simulink model "sim_5_twolink_force_control"  (R2021a)
settings: Solver=VariableStepAuto  StartTime=0.0  StopTime=15  MaxStep=1e-2
values from neighbouring files (symbols this model uses):
  b1 = 0.01    [sim_params.m]    (also in sim_params_force.m)
  b2 = 0.01    [sim_params.m]    (also in sim_params_force.m)
  D = [zeros(n); eye(n)]    [control_comparison_script.m]    (also in gen_twolink_ss.m = reshape([0.0,0.0,0.0,0.0,0.0,0.0,0.0,0.0],[4,2]))
  g = 9.80665    [sim_params.m]    (also in sim_params_force.m)
  L1x = 0.3    [sim_params.m]    (also in sim_params_force.m)
  L1y = 0.050    (= 0.05)    [sim_params.m]    (also in sim_params_force.m)
  L1z = 0.05    [sim_params.m]    (also in sim_params_force.m)
  L2x = 0.15    [sim_params.m]    (also in sim_params_force.m = 0.3)
  L2y = 0.05    [sim_params.m]    (also in sim_params_force.m)
  L2z = 0.05    [sim_params.m]    (also in sim_params_force.m)
  m1 = m1*1.25    [control_comparison_script.m]    (also in sim_params.m = 2.775; sim_params_force.m = 2.775)
  m2 = m2*1.25    [control_comparison_script.m]    (also in sim_params.m = 1.3875; sim_params_force.m = 2.775)
  max_joint_torque1 = 20    [sim_params.m]    (also in sim_params_force.m)
  max_joint_torque2 = 10    [sim_params.m]    (also in sim_params_force.m = 20)
undefined symbols (not defined in the file or in its folder): Da, KD, KD_a, Kd_p, Kd_p2, Kdt, KF, Kf_v, Kf_v2, KI, Ki_f, Ki_f2, Ki_p, Ki_p2, KP, KP_a, Kp_f, Kp_f2, Kp_p, Kp_p2, Levenberg, Ma, Marquardt, R_env, sigbuilder_block, W_env, X, Xenv, Y, Z
libraries: sm_lib x72, nesl_utility x58, pid_lib x14, simulink x3, robotmaniplib x2, robotcorelib x1
(part 6 of 6)

== matlab function sim_5_twolink_force_control/Controller/Hybrid Force//position control /Position Controller1/Position Projection/Position projection (SJ)+ ==
  data: L_1 input; L_2 input; SJ_pinv output; theta_1 input; theta_2 input
function SJ_pinv = P_position(L_1,L_2,theta_1,theta_2)
% Position projection pinv(SJ)
% StJ_t = transpose((1-S)*J)

% position control in y axis
SJ_pinv = [
[0, (L_2*cos((theta_1))*L_1^2 + L_1*cos((theta_1) + (theta_2))*L_2^2)/(L_2^2*cos(theta_1 + theta_2)*L_1^2*cos((theta_1)) + L_1^2*cos(theta_1)*cos((theta_1) + (theta_2))*L_2^2 + L_1*L_2*cos(theta_1)*L_1^2*cos((theta_1)) + 2*L_1*L_2*cos((theta_1) + (theta_2))*cos(theta_1 + theta_2)*L_2^2)]
[0,                                        (L_1*cos((theta_1) + (theta_2))*L_2^2)/(L_2^2*cos(theta_1 + theta_2)*L_1^2*cos((theta_1)) + L_1^2*cos(theta_1)*cos((theta_1) + (theta_2))*L_2^2 + L_1*L_2*cos(theta_1)*L_1^2*cos(theta_1) + 2*L_1*L_2*cos(theta_1 + theta_2)*cos(theta_1 + theta_2)*L_2^2)]
];


% full position control 
% SJ_pinv = [
% [                                 cos(theta_1 + theta_2)/(L_1*sin(theta_2)),                                  sin(theta_1 + theta_2)/(L_1*sin(theta_2))]
% [-(L_2*cos(theta_1 + theta_2) + L_1*cos(theta_1))/(L_1*L_2*sin(theta_2)), -(L_1*sin(theta_1) + L_2*sin(theta_1 + theta_2))/(L_1*L_2*sin(theta_2))]
%     ];

== matlab function sim_5_twolink_force_control/Controller/Hybrid Force//position control /Position Controller1/Position Projection1/Position projection (SJ)+ ==
  data: L_1 input; L_2 input; SJ_pinv output; theta_1 input; theta_2 input
function SJ_pinv = P_position(L_1,L_2,theta_1,theta_2)
% Position projection pinv(SJ)
% StJ_t = transpose((1-S)*J)

% position control in y axis
SJ_pinv = [
[0, (L_2*cos((theta_1))*L_1^2 + L_1*cos((theta_1) + (theta_2))*L_2^2)/(L_2^2*cos(theta_1 + theta_2)*L_1^2*cos((theta_1)) + L_1^2*cos(theta_1)*cos((theta_1) + (theta_2))*L_2^2 + L_1*L_2*cos(theta_1)*L_1^2*cos((theta_1)) + 2*L_1*L_2*cos((theta_1) + (theta_2))*cos(theta_1 + theta_2)*L_2^2)]
[0,                                        (L_1*cos((theta_1) + (theta_2))*L_2^2)/(L_2^2*cos(theta_1 + theta_2)*L_1^2*cos((theta_1)) + L_1^2*cos(theta_1)*cos((theta_1) + (theta_2))*L_2^2 + L_1*L_2*cos(theta_1)*L_1^2*cos(theta_1) + 2*L_1*L_2*cos(theta_1 + theta_2)*cos(theta_1 + theta_2)*L_2^2)]
];


% full position control 
% SJ_pinv = [
% [                                 cos(theta_1 + theta_2)/(L_1*sin(theta_2)),                                  sin(theta_1 + theta_2)/(L_1*sin(theta_2))]
% [-(L_2*cos(theta_1 + theta_2) + L_1*cos(theta_1))/(L_1*L_2*sin(theta_2)), -(L_1*sin(theta_1) + L_2*sin(theta_1 + theta_2))/(L_1*L_2*sin(theta_2))]
%     ];

== matlab function sim_5_twolink_force_control/Controller/Hybrid Force//position control /Force Controller/Force Projection1/Force projection (StJ_t) ==
  data: L_1 input; L_2 input; StJ_t output; theta_1 input; theta_2 input
function StJ_t = P_force(L_1,L_2,theta_1,theta_2)
% Force projection (StJ_t)
% StJ_t = transpose((1-S)*J)

% force control in X axis
StJ_t = [
    [- L_1*sin(theta_1) - L_2*sin(theta_1 + theta_2), 0]
    [                    -L_2*sin(theta_1 + theta_2), 0]
];

% no force control at all

% StJ_t = [
%     0   0;
%     0   0;
% ];

== matlab function sim_5_twolink_force_control/Controller/Hybrid Force//position control /Force Controller/Force Projection2/Force projection (StJ_t) ==
  data: L_1 input; L_2 input; StJ_t output; theta_1 input; theta_2 input
function StJ_t = P_force(L_1,L_2,theta_1,theta_2)
% Force projection (StJ_t)
% StJ_t = transpose((1-S)*J)

% force control in X axis
StJ_t = [
    [- L_1*sin(theta_1) - L_2*sin(theta_1 + theta_2), 0]
    [                    -L_2*sin(theta_1 + theta_2), 0]
];

% no force control at all

% StJ_t = [
%     0   0;
%     0   0;
% ];

== matlab function sim_5_twolink_force_control/Controller/Hybrid Force//position control /Jacobian/Jacobian ==
  data: L_1 input; J output; L_2 input; theta_1 input; theta_2 input
function J = jacobian_geom(L_1,L_2,theta_1,theta_2)

J = [
       -L_1.*sin(theta_1)-L_2.*sin(theta_1+theta_2) , -L_2.*sin(theta_1+theta_2) ;
        L_1.*cos(theta_1)+L_2.*cos(theta_1+theta_2) ,  L_2.*cos(theta_1+theta_2) ;
    ];

== matlab function sim_5_twolink_force_control/Controller/Hybrid Force//position control (stiff)/Force Controller/Force Projection/Force projection (StJ_t) ==
  data: L_1 input; L_2 input; StJ_t output; theta_1 input; theta_2 input
function StJ_t = P_force(L_1,L_2,theta_1,theta_2)
% Force projection (StJ_t)
% StJ_t = transpose((1-S)*J)

% force control in X axis
StJ_t = [
    [- L_1*sin(theta_1) - L_2*sin(theta_1 + theta_2), 0]
    [                    -L_2*sin(theta_1 + theta_2), 0]
];

% no force control at all

% StJ_t = [
%     0   0;
%     0   0;
% ];

== matlab function sim_5_twolink_force_control/Controller/Hybrid Force//position control (stiff)/Force Controller/Force Projection1/Force projection (StJ_t) ==
  data: L_1 input; L_2 input; StJ_t output; theta_1 input; theta_2 input
function StJ_t = P_force(L_1,L_2,theta_1,theta_2)
% Force projection (StJ_t)
% StJ_t = transpose((1-S)*J)

% force control in X axis
StJ_t = [
    [- L_1*sin(theta_1) - L_2*sin(theta_1 + theta_2), 0]
    [                    -L_2*sin(theta_1 + theta_2), 0]
];

% no force control at all

% StJ_t = [
%     0   0;
%     0   0;
% ];

== matlab function sim_5_twolink_force_control/Controller/Hybrid Force//position control (stiff)/Force Controller/Force Projection2/Force projection (StJ_t) ==
  data: L_1 input; L_2 input; StJ_t output; theta_1 input; theta_2 input
function StJ_t = P_force(L_1,L_2,theta_1,theta_2)
% Force projection (StJ_t)
% StJ_t = transpose((1-S)*J)

% force control in X axis
StJ_t = [
    [- L_1*sin(theta_1) - L_2*sin(theta_1 + theta_2), 0]
    [                    -L_2*sin(theta_1 + theta_2), 0]
];

% no force control at all

% StJ_t = [
%     0   0;
%     0   0;
% ];

== matlab function sim_5_twolink_force_control/Controller/Hybrid Force//position control (stiff)/Jacobian/Jacobian ==
  data: L_1 input; J output; L_2 input; theta_1 input; theta_2 input
function J = jacobian_geom(L_1,L_2,theta_1,theta_2)

J = [
       -L_1.*sin(theta_1)-L_2.*sin(theta_1+theta_2) , -L_2.*sin(theta_1+theta_2) ;
        L_1.*cos(theta_1)+L_2.*cos(theta_1+theta_2) ,  L_2.*cos(theta_1+theta_2) ;
    ];

== matlab function sim_5_twolink_force_control/Forward Kinmatics/Jacobian/Jacobian ==
  data: L_1 input; J output; L_2 input; theta_1 input; theta_2 input
function J = jacobian_geom(L_1,L_2,theta_1,theta_2)

J = [
       -L_1.*sin(theta_1)-L_2.*sin(theta_1+theta_2) , -L_2.*sin(theta_1+theta_2) ;
        L_1.*cos(theta_1)+L_2.*cos(theta_1+theta_2) ,  L_2.*cos(theta_1+theta_2) ;
    ];

== matlab function sim_5_twolink_force_control/Controller/Hybrid Force//position control (stiff)/Position Controller1/Position Projection/Position projection (SJ)+ ==
  data: L_1 input; L_2 input; SJ_pinv output; theta_1 input; theta_2 input
function SJ_pinv = P_position(L_1,L_2,theta_1,theta_2)
% Position projection pinv(SJ)
% StJ_t = transpose((1-S)*J)

% position control in y axis
SJ_pinv = [
[0, (L_2*cos((theta_1))*L_1^2 + L_1*cos((theta_1) + (theta_2))*L_2^2)/(L_2^2*cos(theta_1 + theta_2)*L_1^2*cos((theta_1)) + L_1^2*cos(theta_1)*cos((theta_1) + (theta_2))*L_2^2 + L_1*L_2*cos(theta_1)*L_1^2*cos((theta_1)) + 2*L_1*L_2*cos((theta_1) + (theta_2))*cos(theta_1 + theta_2)*L_2^2)]
[0,                                        (L_1*cos((theta_1) + (theta_2))*L_2^2)/(L_2^2*cos(theta_1 + theta_2)*L_1^2*cos((theta_1)) + L_1^2*cos(theta_1)*cos((theta_1) + (theta_2))*L_2^2 + L_1*L_2*cos(theta_1)*L_1^2*cos(theta_1) + 2*L_1*L_2*cos(theta_1 + theta_2)*cos(theta_1 + theta_2)*L_2^2)]
];


% full position control 
% SJ_pinv = [
% [                                 cos(theta_1 + theta_2)/(L_1*sin(theta_2)),                                  sin(theta_1 + theta_2)/(L_1*sin(theta_2))]
% [-(L_2*cos(theta_1 + theta_2) + L_1*cos(theta_1))/(L_1*L_2*sin(theta_2)), -(L_1*sin(theta_1) + L_2*sin(theta_1 + theta_2))/(L_1*L_2*sin(theta_2))]
%     ];

== matlab function sim_5_twolink_force_control/Controller/Hybrid Force//position control (stiff)/Position Controller1/Position Projection1/Position projection (SJ)+ ==
  data: L_1 input; L_2 input; SJ_pinv output; theta_1 input; theta_2 input
function SJ_pinv = P_position(L_1,L_2,theta_1,theta_2)
% Position projection pinv(SJ)
% StJ_t = transpose((1-S)*J)

% position control in y axis
SJ_pinv = [
[0, (L_2*cos((theta_1))*L_1^2 + L_1*cos((theta_1) + (theta_2))*L_2^2)/(L_2^2*cos(theta_1 + theta_2)*L_1^2*cos((theta_1)) + L_1^2*cos(theta_1)*cos((theta_1) + (theta_2))*L_2^2 + L_1*L_2*cos(theta_1)*L_1^2*cos((theta_1)) + 2*L_1*L_2*cos((theta_1) + (theta_2))*cos(theta_1 + theta_2)*L_2^2)]
[0,                                        (L_1*cos((theta_1) + (theta_2))*L_2^2)/(L_2^2*cos(theta_1 + theta_2)*L_1^2*cos((theta_1)) + L_1^2*cos(theta_1)*cos((theta_1) + (theta_2))*L_2^2 + L_1*L_2*cos(theta_1)*L_1^2*cos(theta_1) + 2*L_1*L_2*cos(theta_1 + theta_2)*cos(theta_1 + theta_2)*L_2^2)]
];


% full position control 
% SJ_pinv = [
% [                                 cos(theta_1 + theta_2)/(L_1*sin(theta_2)),                                  sin(theta_1 + theta_2)/(L_1*sin(theta_2))]
% [-(L_2*cos(theta_1 + theta_2) + L_1*cos(theta_1))/(L_1*L_2*sin(theta_2)), -(L_1*sin(theta_1) + L_2*sin(theta_1 + theta_2))/(L_1*L_2*sin(theta_2))]
%     ];
